simulink model "HPP_IMV_18_1"  (R2018a)
settings: Solver=FixedStepDiscrete  StartTime=0.0  StopTime=10.0  RelTol=1e-3
settings Model: Creator=Sohan  LastModifiedBy=Sohan
settings ConfigComp: DVTestSuiteOptimization=CombinedObjectives (Nonlinear Extended)  DVDetectDeadLogic=on  DVDetectFloatOverflow=off

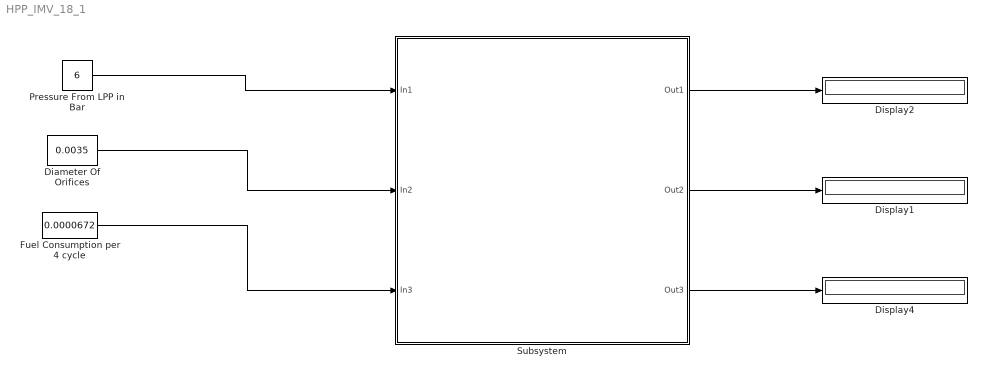
== system HPP_IMV_18_1 ==
  Diameter Of Orifices : Constant  Value=0.0035  OutDataTypeStr=fixdt(1,16,23)
  Display1 : Display
      settings: Format=bank
  Display2 : Display
      settings: Format=bank
  Display4 : Display
  Fuel Consumption per 4 cycle : Constant  Value=0.0000672
  Pressure From LPP in Bar : Constant  Value=6  OutDataTypeStr=uint8
  Subsystem : Subsystem  TreatAsAtomicUnit=on
  wires:
  Pressure From LPP in Bar/1 -> Subsystem/1(In1)
  Diameter Of Orifices/1 -> Subsystem/2(In2)
  Fuel Consumption per 4 cycle/1 -> Subsystem/3(In3)
  Subsystem/1(Out1) -> Display2/1
  Subsystem/2(Out2) -> Display1/1
  Subsystem/3(Out3) -> Display4/1

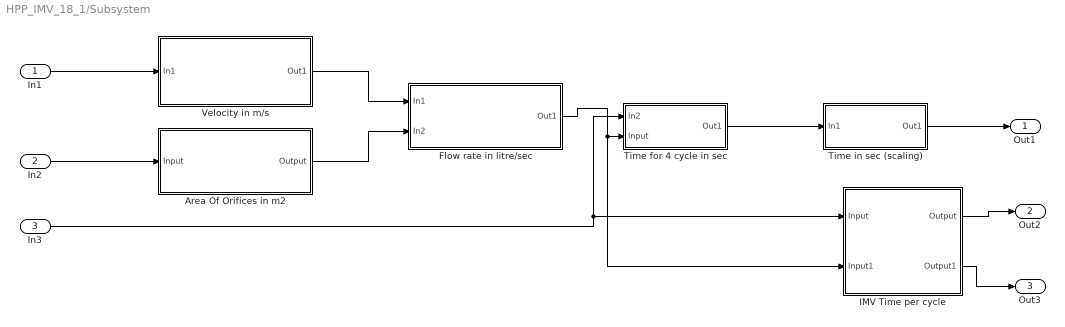
== system HPP_IMV_18_1/Subsystem ==
  In1 : Inport
  In2 : Inport  Port=2
  In3 : Inport  Port=3
  Area Of Orifices in m2 : Subsystem
  Flow rate in litre/sec : Subsystem
  IMV Time per cycle : Subsystem
  Time for 4 cycle in sec : Subsystem
  Time in sec (scaling) : Subsystem
  Velocity in m/s : Subsystem
  Out1 : Outport
  Out2 : Outport  Port=2
  Out3 : Outport  Port=3
  wires:
  IMV Time per cycle/2(Output1) -> Out3/1
  Area Of Orifices in m2/1(Output) -> Flow rate in litre/sec/2(In2)
  Flow rate in litre/sec/1(Out1) -> Time for 4 cycle in sec/2(Input), IMV Time per cycle/2(Input1)
  In1/1 -> Velocity in m/s/1(In1)
  Velocity in m/s/1(Out1) -> Flow rate in litre/sec/1(In1)
  In3/1 -> Time for 4 cycle in sec/1(In2), IMV Time per cycle/1(Input)
  Time for 4 cycle in sec/1(Out1) -> Time in sec (scaling)/1(In1)
  IMV Time per cycle/1(Output) -> Out2/1
  Time in sec (scaling)/1(Out1) -> Out1/1
  In2/1 -> Area Of Orifices in m2/1(Input)

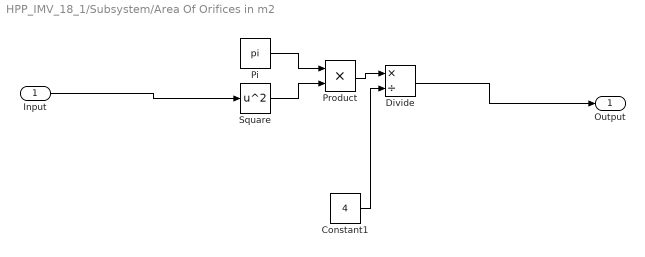
== system HPP_IMV_18_1/Subsystem/Area Of Orifices in m2 ==
  Input : Inport
  Constant1 : Constant  Value=4
  Divide : Product  Inputs=*/
  Pi : Constant  Value=pi
  Product : Product
  Square : Math  Operator=square  SaturateOnIntegerOverflow=on
  Output : Outport
  wires:
  Input/1 -> Square/1
  Pi/1 -> Product/1
  Square/1 -> Product/2
  Product/1 -> Divide/1
  Constant1/1 -> Divide/2
  Divide/1 -> Output/1

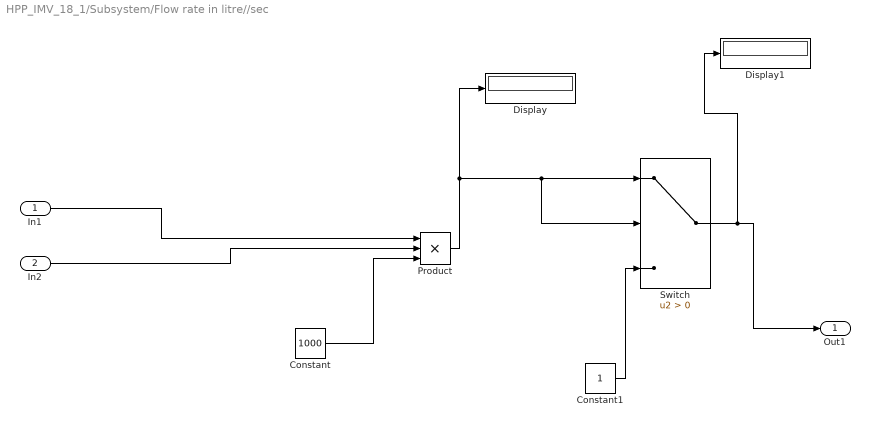
== system HPP_IMV_18_1/Subsystem/Flow rate in litre//sec ==
  In1 : Inport
  In2 : Inport  Port=2
  Constant : Constant  Value=1000
  Constant1 : Constant
  Display : Display
  Display1 : Display
  Product : Product  Inputs=3
  Switch : Switch  Criteria=u2 > Threshold
  Out1 : Outport
  wires:
  In2/1 -> Product/2
  In1/1 -> Product/1
  Constant/1 -> Product/3
  Switch/1 -> Display1/1, Out1/1
  Product/1 -> Switch/2, Switch/1, Display/1
  Constant1/1 -> Switch/3

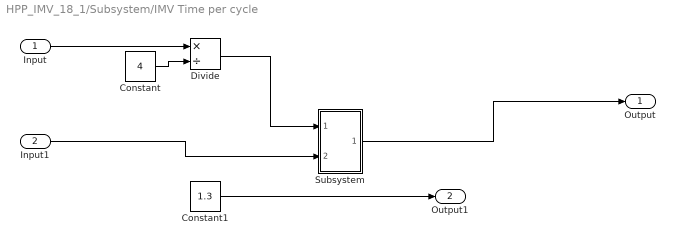
== system HPP_IMV_18_1/Subsystem/IMV Time per cycle ==
  Input : Inport
  Input1 : Inport  Port=2
  Constant : Constant  Value=4
  Constant1 : Constant  Value=1.3
  Divide : Product  Inputs=*/
  Subsystem : Subsystem
  Output : Outport
  Output1 : Outport  Port=2
  wires:
  Input/1 -> Divide/1
  Input1/1 -> Subsystem/2(In2)
  Subsystem/1(Out1) -> Output/1
  Divide/1 -> Subsystem/1(In1)
  Constant/1 -> Divide/2
  Constant1/1 -> Output1/1

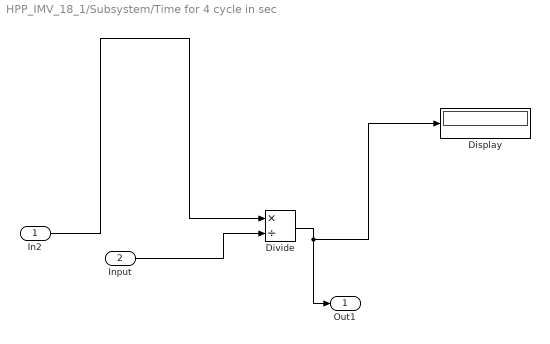
== system HPP_IMV_18_1/Subsystem/Time for 4 cycle in sec ==
  In2 : Inport
  Input : Inport  Port=2
  Display : Display
  Divide : Product  Inputs=*/
  Out1 : Outport
  wires:
  Divide/1 -> Display/1, Out1/1
  In2/1 -> Divide/1
  Input/1 -> Divide/2

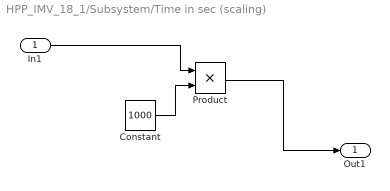
== system HPP_IMV_18_1/Subsystem/Time in sec (scaling) ==
  In1 : Inport
  Constant : Constant  Value=1000
  Product : Product
  Out1 : Outport
  wires:
  In1/1 -> Product/1
  Product/1 -> Out1/1
  Constant/1 -> Product/2

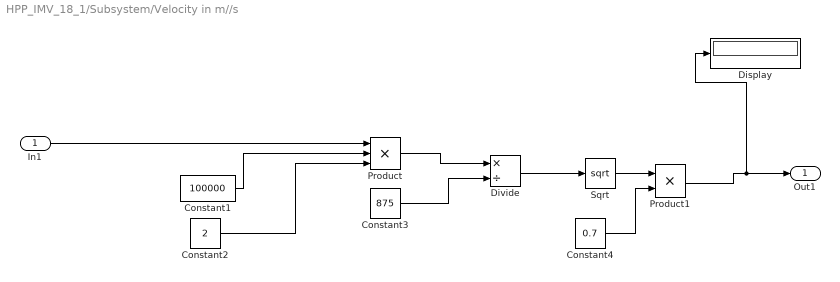
== system HPP_IMV_18_1/Subsystem/Velocity in m//s ==
  In1 : Inport
  Constant1 : Constant  Value=100000
  Constant2 : Constant  Value=2
  Constant3 : Constant  Value=875
  Constant4 : Constant  Value=0.7
  Display : Display
  Divide : Product  Inputs=*/
  Product : Product  Inputs=3
  Product1 : Product
  Sqrt : Sqrt  SaturateOnIntegerOverflow=on
  Out1 : Outport
  wires:
  In1/1 -> Product/1
  Constant3/1 -> Divide/2
  Constant1/1 -> Product/2
  Product/1 -> Divide/1
  Constant4/1 -> Product1/2
  Sqrt/1 -> Product1/1
  Product1/1 -> Display/1, Out1/1
  Constant2/1 -> Product/3
  Divide/1 -> Sqrt/1

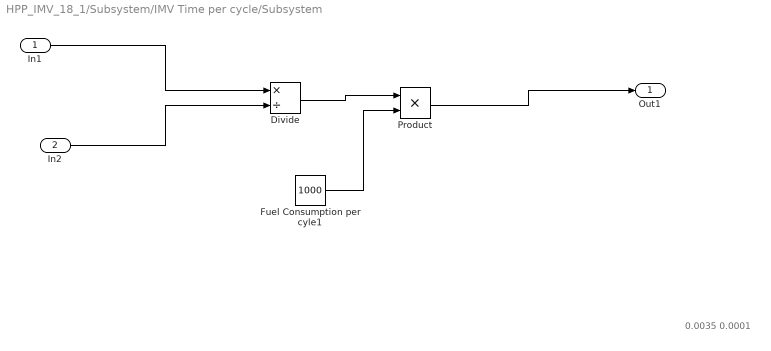
== system HPP_IMV_18_1/Subsystem/IMV Time per cycle/Subsystem ==
  note: 0.0035
      | 0.0001
  In1 : Inport
  In2 : Inport  Port=2
  Divide : Product  Inputs=*/
  Fuel Consumption per cyle1 : Constant  Value=1000
  Product : Product
  Out1 : Outport
  wires:
  Divide/1 -> Product/1
  In2/1 -> Divide/2
  Fuel Consumption per cyle1/1 -> Product/2
  Product/1 -> Out1/1
  In1/1 -> Divide/1
